simulink model "a2024_V2X_6V_Simulink_model"  (R2023b)
settings: Solver=VariableStepAuto  StartTime=0.0  StopTime=30  MaxStep=1e-2  RelTol=1e-3  AbsTol=1e-3
values from neighbouring files (symbols this model uses):
  b = 1.6    [a2024_v2x_matlab_6veh.m]
  mEgo = 1500    [a2024_v2x_matlab_6veh.m]
  Mode = 1    [a2024_v2x_matlab_6veh.m]    (also in v2x_matlab.m; v2x_matlabV2.m; v2x_matlab_6veh.m; v2x_matlab_R.m)
  pilot = (randi(s,[0 1],pilotsPerSym,1)-0.5)*2    [v2x_matlab.m]
  RxPowerV1 = zeros(sizeEgoWP+2, sizeV1WP+2)    [a2024_v2x_matlab_6veh.m]
  RxPowerV2 = zeros(sizeEgoWP+2, sizeV2WP+2)    [a2024_v2x_matlab_6veh.m]
  RxPowerV3 = zeros(sizeEgoWP+2, sizeV3WP+2)    [a2024_v2x_matlab_6veh.m]
  RxPowerV4 = zeros(sizeEgoWP+2, sizeV4WP+2)    [a2024_v2x_matlab_6veh.m]
  RxPowerV5 = zeros(sizeEgoWP+2, sizeV5WP+2)    [a2024_v2x_matlab_6veh.m]
  RxPowerV6 = zeros(sizeEgoWP+2, sizeV6WP+2)    [a2024_v2x_matlab_6veh.m]
  sampleTime = 0.1    [a2024_v2x_matlab_6veh.m]    (also in v2x_matlab.m; v2x_matlabV2.m; v2x_matlab_6veh.m; v2x_matlab_R.m)
  t_gap = 1.4    [a2024_v2x_matlab_6veh.m]
  waypoints = [egoWP(:,2) egoWP(:,1), zeroforwp]    [a2024_v2x_matlab_6veh.m]    (also in misc.m = data.data.ActorSpecifications(1,1).Waypoints(:,[1,2]); v2x_matlab.m = data.data.ActorSpecifications(1,1).Waypoints(:,[1,2]); v2x_matlabV2.m = [5 -1.6 0; v2x_matlab_R.m = [5 -1.6 0)
  ZeroActors = struct(     'ActorID',0,     'Position', [1000 1000 1000],      'Velocity', [0 0 0],      'Roll', 0,      'Pitch', 0,      'Yaw', 0,      'AngularVelocity', [0 0 0])    [v2x_matlabV2.m]    (also in v2x_matlab_R.m)
undefined symbols (not defined in the file or in its folder): driving, PredictionHorizon, Ts
libraries: commofdm x50, commcnvcod2 x39, simulink x34, commdigbbndam3 x31, commblkintrlv2 x26, commdigbbndpm3 x14, simulink_extras x12, drivingscenarioandsensors x3, mpcadaslib x2, commchan3 x1, vehdynlibdriver x1, commrandsrc3 x1
(part 3 of 6)

== system a2024_V2X_6V_Simulink_model/Subsystem/1//2 64 QAM ==
  Bits : Inport
  Pilot : Inport  Port=2
  Constant2 : Constant  Value=[zeros(887,1)]  VectorParams1D=off  SampleTime=-1
  Convolutional Encoder : commcnvcod2/Convolutional Encoder  trellis=poly2trellis(7, [171 133])  opMode=Truncated (reset every frame)  DelayedResetAction=on  hasIniStPort=off  hasFinStPort=off  usePuncVector=off  punctureVector=[1;1;0;1;1;0;1;1;0;1;0;1;1;0;1;1;0;1]  reset=Unused parameter value
      settings: LibrarySourceBlock=|
      | commhdlcnvcod/Convolutional
      | Encoder
  Display : Display
  OFDM Modulator1 : commofdm/OFDM Modulator  StatePerturbationForJacobian=1.0e-05  FFTLength=1024  NumGuardBandCarriers=[0;0]  InsertDCNull=on  PilotInputPort=on  PilotCarrierIndices=pilotInd  CyclicPrefixLength=512  Windowing=off  WindowLength=16  OversamplingFactor=1  NumSymbols=1  NumTransmitAntennas=1  SimulateUsing=Interpreted execution
  Rectangular QAM Modulator Baseband2 : commdigbbndam3/Rectangular QAM Modulator Baseband  M=2^6  InType=Bit  Enc=Gray  Mapping=[0:15]  PowType=Average Power  MinDist=2  AvgPow=42  PeakPow=1  Ph=0  outDtype=double  outWordLen=16  outUDDataType=sfix(16)  outFracLenMode=Best precision  outFracLen=15  outDataTypeStr=double  outLastDataTypeStr=double
      settings: LibrarySourceBlock=|
      | commhdldigbbndam/Rectangular QAM
      | Modulator
      | Baseband
  Vector Concatenate : Concatenate
  Modulated : Outport
  wires:
  Bits/1 -> Convolutional Encoder/1  "Raw"
  Vector Concatenate/1 -> OFDM Modulator1/1  "After QAM Mod"
  Constant2/1 -> Vector Concatenate/2
  Convolutional Encoder/1 -> Rectangular QAM Modulator Baseband2/1, Display/1  "Before QAM"
  OFDM Modulator1/1 -> Modulated/1  "Sent"
  Pilot/1 -> OFDM Modulator1/2
  Rectangular QAM Modulator Baseband2/1 -> Vector Concatenate/1  "Before OFDM"

== system a2024_V2X_6V_Simulink_model/Subsystem/1//2 QPSK ==
  Bits : Inport
  Pilot : Inport  Port=2
  Constant2 : Constant  Commented=on  Value=[zeros(695,1)]  VectorParams1D=off  SampleTime=-1
  Convolutional Encoder : commcnvcod2/Convolutional Encoder  trellis=poly2trellis(7, [171 133])  opMode=Truncated (reset every frame)  DelayedResetAction=on  hasIniStPort=off  hasFinStPort=off  usePuncVector=on  punctureVector=[1;1]  reset=Unused parameter value
      settings: LibrarySourceBlock=|
      | commhdlcnvcod/Convolutional
      | Encoder
  Gain : Gain  Gain=1/sqrt(10)
  Matrix Concatenate : Concatenate  NumInputs=6  Mode=Multidimensional array  ConcatenateDimension=2
  OFDM Modulator1 : commofdm/OFDM Modulator  StatePerturbationForJacobian=1.0e-05  FFTLength=64  NumGuardBandCarriers=[6;5]  InsertDCNull=on  PilotInputPort=on  PilotCarrierIndices=[12; 26; 40; 54]  CyclicPrefixLength=16  Windowing=off  WindowLength=16  OversamplingFactor=1  NumSymbols=6  NumTransmitAntennas=1  SimulateUsing=Interpreted execution
  QPSK Modulator Baseband : commdigbbndpm3/QPSK Modulator Baseband  InType=Bit  Enc=Gray  Ph=pi/4  outDtype=double  outWordLen=16  outUDDataType=sfix(16)  outFracLenMode=Best precision  outFracLen=15  outDataTypeStr=double  outLastDataTypeStr=double
      settings: LibrarySourceBlock=|
      | commhdldigbbndpm/QPSK
      | Modulator
      | Baseband
  Random Interleaver : commblkintrlv2/Random Interleaver  StatePerturbationForJacobian=1.0e-05  N=576  seed=12345
  Reshape : Reshape  OutputDimensionality=Customize  OutputDimensions=[48,6]
  Vector Concatenate : Concatenate  Commented=on
  Modulated : Outport
  wires:
  OFDM Modulator1/1 -> Modulated/1  "OFDM modulated"
  QPSK Modulator Baseband/1 -> Gain/1
  Bits/1 -> Convolutional Encoder/1
  Convolutional Encoder/1 -> Random Interleaver/1
  Gain/1 -> Reshape/1  "After QAM Mod"
  Pilot/1 -> Matrix Concatenate/1, Matrix Concatenate/2, Matrix Concatenate/3, Matrix Concatenate/6, Matrix Concatenate/5, Matrix Concatenate/4
  Random Interleaver/1 -> QPSK Modulator Baseband/1
  Reshape/1 -> OFDM Modulator1/1
  Constant2/1 -> Vector Concatenate/2
  Matrix Concatenate/1 -> OFDM Modulator1/2

== system a2024_V2X_6V_Simulink_model/Subsystem/3//4 64 QAM ==
  Bits : Inport
  Pilot : Inport  Port=2
  Constant2 : Constant  Value=[zeros(32,1)']  VectorParams1D=off  SampleTime=-1
  Convolutional Encoder : commcnvcod2/Convolutional Encoder  trellis=poly2trellis(7, [171 133])  opMode=Truncated (reset every frame)  DelayedResetAction=on  hasIniStPort=off  hasFinStPort=off  usePuncVector=on  punctureVector=[1;1;0;1;1;0]  reset=Unused parameter value
      settings: LibrarySourceBlock=|
      | commhdlcnvcod/Convolutional
      | Encoder
  Display : Display
  Matrix Concatenate : Concatenate  Mode=Multidimensional array  ConcatenateDimension=2
  OFDM Modulator1 : commofdm/OFDM Modulator  StatePerturbationForJacobian=1.0e-05  FFTLength=64  NumGuardBandCarriers=[6;5]  InsertDCNull=on  PilotInputPort=on  PilotCarrierIndices=[12; 26; 40; 54]  CyclicPrefixLength=16  Windowing=off  WindowLength=16  OversamplingFactor=1  NumSymbols=2  NumTransmitAntennas=1  SimulateUsing=Interpreted execution
  Random Interleaver : commblkintrlv2/Random Interleaver  StatePerturbationForJacobian=1.0e-05  N=384  seed=12345
  Rectangular QAM Modulator Baseband2 : commdigbbndam3/Rectangular QAM Modulator Baseband  M=2^6  InType=Bit  Enc=Gray  Mapping=[0:15]  PowType=Average Power  MinDist=2  AvgPow=0.1  PeakPow=1  Ph=0  outDtype=double  outWordLen=16  outUDDataType=sfix(16)  outFracLenMode=Best precision  outFracLen=15  outDataTypeStr=double  outLastDataTypeStr=double
      settings: LibrarySourceBlock=|
      | commhdldigbbndam/Rectangular QAM
      | Modulator
      | Baseband
  Reshape : Reshape  OutputDimensionality=Customize  OutputDimensions=[48,2]
  Vector Concatenate : Concatenate
  Modulated : Outport
  wires:
  Rectangular QAM Modulator Baseband2/1 -> Vector Concatenate/1  "Before OFDM"
  OFDM Modulator1/1 -> Modulated/1  "Sent"
  Convolutional Encoder/1 -> Random Interleaver/1  "Before QAM"
  Constant2/1 -> Vector Concatenate/2
  Vector Concatenate/1 -> Reshape/1  "After QAM Mod"
  Bits/1 -> Convolutional Encoder/1  "Raw"
  Random Interleaver/1 -> Display/1, Rectangular QAM Modulator Baseband2/1
  Reshape/1 -> OFDM Modulator1/1
  Pilot/1 -> Matrix Concatenate/1, Matrix Concatenate/2
  Matrix Concatenate/1 -> OFDM Modulator1/2

== system a2024_V2X_6V_Simulink_model/Subsystem10/1//2 64 QAM1 ==
  Output : Inport
  Bit to Integer Converter2 : simulink/Logic and Bit Operations/Bit to Integer Converter  nbits=16  bitOrder=MSB first  signedOutputValues=Signed  outDtype=int16  outDtypeSigned=int16
  Complex to Real-Imag : ComplexToRealImag
  Display : Display
  Display2 : Display
  OFDM Demodulator : commofdm/OFDM Demodulator  StatePerturbationForJacobian=1.0e-05  FFTLength=1024  NumGuardBandCarriers=[0; 0]  RemoveDCCarrier=on  PilotOutputPort=on  PilotCarrierIndices=pilotInd  CyclicPrefixLength=512  OversamplingFactor=1  NumSymbols=1  NumReceiveAntennas=1  SimulateUsing=Interpreted execution
  Rectangular QAM Demodulator Baseband2 : commdigbbndam3/Rectangular QAM Demodulator Baseband  M=64  OutType=Bit  DecType=Hard decision  VarSource=Dialog  Variance=1  Dec=Gray  Mapping=[0:15]  PowType=Average Power  MinDist=2  AvgPow=42  PeakPow=1  Ph=0  outDtype1=int16  outDtype2=int16  derotateFactorWordLen=16  derotateFactorDataTypeStr=Inherit: Same word length as input  derotateFactorLastDataTypeStr=Inherit: Same word length as input  denormFactorWordLen=16  denormFactorDataTypeStr=Inherit: Same word length as input  denormFactorLastDataTypeStr=Inherit: Same word length as input  prodOutWordLen=32  prodOutOverflowMode=Wrap  prodOutRoundingMode=Floor  prodOutOvFlMode=off  prodOutOvFlModeLastStrValue=off  sumWordLen=32
      settings: LibrarySourceBlock=|
      | commhdldigbbndam/Rectangular QAM
      | Demodulator
      | Baseband
  Selector : Selector  InputPortWidth=983  IndexOptions=Index vector (dialog)  Indices=[1:96]  OutputSizes=1
  Selector1 : Selector  Commented=on  InputPortWidth=18  IndexOptions=Index vector (dialog)  Indices=[7:18]  OutputSizes=1
  Selector2 : Selector  Commented=on  InputPortWidth=18  IndexOptions=Index vector (dialog)  Indices=[1:6]  OutputSizes=1
  Vector Concatenate : Concatenate  Commented=on
  Viterbi Decoder : commcnvcod2/Viterbi Decoder  trellis=poly2trellis(7, [171 133])  isPunctured=off  punctureVector=[1;1;0;1;1;0;1;1;0;1;0;1;1;0;1;1;0;1]  erasures=off  dectype=Hard decision  nsdecb=4  runSigValErrCheck=off  tbdepth=96  opmode=Truncated  reset=off  delayedResetAction=on  smWordLength=16  outDataType=int16
      settings: LibrarySourceBlock=commhdlcnvcod/Viterbi Decoder
  Modulated : Outport
  wires:
  OFDM Demodulator/2 -> Complex to Real-Imag/1
  Output/1 -> OFDM Demodulator/1  "Sent"
  Selector/1 -> Rectangular QAM Demodulator Baseband2/1  "After OFDM"
  Viterbi Decoder/1 -> Bit to Integer Converter2/1  "Raw"
  OFDM Demodulator/1 -> Selector/1  "After OFDM"
  Rectangular QAM Demodulator Baseband2/1 -> Viterbi Decoder/1  "After QAM"
  Complex to Real-Imag/1 -> Display/1
  Bit to Integer Converter2/1 -> Display2/1, Modulated/1
  Selector1/1 -> Vector Concatenate/1
  Selector2/1 -> Vector Concatenate/2

== system a2024_V2X_6V_Simulink_model/Subsystem10/1//2 QPSK ==
  Output : Inport
  Bit to Integer Converter2 : simulink/Logic and Bit Operations/Bit to Integer Converter  nbits=16  bitOrder=MSB first  signedOutputValues=Signed  outDtype=int16  outDtypeSigned=int16
  Display : Display
  OFDM Demodulator1 : commofdm/OFDM Demodulator  Commented=on  StatePerturbationForJacobian=1.0e-05  FFTLength=64  NumGuardBandCarriers=[0; 0]  RemoveDCCarrier=on  PilotOutputPort=on  PilotCarrierIndices=[12; 26; 40; 54]  CyclicPrefixLength=32  OversamplingFactor=3  NumSymbols=1  NumReceiveAntennas=1  SimulateUsing=Interpreted execution
  OFDM Demodulator2 : commofdm/OFDM Demodulator  StatePerturbationForJacobian=1.0e-05  FFTLength=64  NumGuardBandCarriers=[6; 5]  RemoveDCCarrier=on  PilotOutputPort=on  PilotCarrierIndices=[12; 26; 40; 54]  CyclicPrefixLength=16  OversamplingFactor=1  NumSymbols=6  NumReceiveAntennas=1  SimulateUsing=Interpreted execution
  QPSK Demodulator Baseband : commdigbbndpm3/QPSK Demodulator Baseband  OutType=Bit  DecType=Hard decision  VarSource=Dialog  Variance=1  Dec=Gray  Ph=pi/4  outDtype1=Inherit via internal rule  outDtype2=Inherit via internal rule  derotateFactorWordLen=16  derotateFactorDataTypeStr=Inherit: Same word length as input  derotateFactorLastDataTypeStr=Inherit: Same word length as input
      settings: LibrarySourceBlock=|
      | commhdldigbbndpm/QPSK
      | Demodulator
      | Baseband
  Random Deinterleaver : commblkintrlv2/Random Deinterleaver  StatePerturbationForJacobian=1.0e-05  N=576  seed=12345
  Reshape : Reshape
  Selector : Selector  InputPortWidth=288  IndexOptions=Index vector (dialog)  Indices=[1:288]  OutputSizes=1
  Viterbi Decoder : commcnvcod2/Viterbi Decoder  trellis=poly2trellis(7, [171 133])  isPunctured=on  punctureVector=[1; 1]  erasures=off  dectype=Hard decision  nsdecb=4  runSigValErrCheck=off  tbdepth=30  opmode=Truncated  reset=off  delayedResetAction=on  smWordLength=16  outDataType=Smallest unsigned integer
      settings: LibrarySourceBlock=commhdlcnvcod/Viterbi Decoder
  Modulated : Outport
  wires:
  Random Deinterleaver/1 -> Viterbi Decoder/1
  Reshape/1 -> Selector/1
  Viterbi Decoder/1 -> Bit to Integer Converter2/1
  Bit to Integer Converter2/1 -> Modulated/1
  Selector/1 -> QPSK Demodulator Baseband/1
  QPSK Demodulator Baseband/1 -> Random Deinterleaver/1
  Output/1 -> OFDM Demodulator2/1
  OFDM Demodulator2/1 -> Reshape/1  "Before QAM Demod"
  OFDM Demodulator2/2 -> Display/1

== system a2024_V2X_6V_Simulink_model/Subsystem10/3//4 64 QAM ==
  Output : Inport
  Bit to Integer Converter2 : simulink/Logic and Bit Operations/Bit to Integer Converter  nbits=16  bitOrder=MSB first  signedOutputValues=Signed  outDtype=int16  outDtypeSigned=int16
  Complex to Real-Imag : ComplexToRealImag
  Display : Display
  Display1 : Display
  Display2 : Display
  OFDM Demodulator : commofdm/OFDM Demodulator  StatePerturbationForJacobian=1.0e-05  FFTLength=64  NumGuardBandCarriers=[6; 5]  RemoveDCCarrier=on  PilotOutputPort=on  PilotCarrierIndices=[12; 26; 40; 54]  CyclicPrefixLength=16  OversamplingFactor=1  NumSymbols=2  NumReceiveAntennas=1  SimulateUsing=Interpreted execution
  Random Deinterleaver : commblkintrlv2/Random Deinterleaver  StatePerturbationForJacobian=1.0e-05  N=384  seed=12345
  Rectangular QAM Demodulator Baseband2 : commdigbbndam3/Rectangular QAM Demodulator Baseband  M=64  OutType=Bit  DecType=Hard decision  VarSource=Dialog  Variance=1  Dec=Gray  Mapping=[0:15]  PowType=Average Power  MinDist=2  AvgPow=0.1  PeakPow=1  Ph=0  outDtype1=int16  outDtype2=int16  derotateFactorWordLen=16  derotateFactorDataTypeStr=Inherit: Same word length as input  derotateFactorLastDataTypeStr=Inherit: Same word length as input  denormFactorWordLen=16  denormFactorDataTypeStr=Inherit: Same word length as input  denormFactorLastDataTypeStr=Inherit: Same word length as input  prodOutWordLen=32  prodOutOverflowMode=Wrap  prodOutRoundingMode=Floor  prodOutOvFlMode=off  prodOutOvFlModeLastStrValue=off  sumWordLen=32
      settings: LibrarySourceBlock=|
      | commhdldigbbndam/Rectangular QAM
      | Demodulator
      | Baseband
  Reshape : Reshape
  Selector : Selector  InputPortWidth=96  IndexOptions=Index vector (dialog)  Indices=[1:64]  OutputSizes=1
  Selector1 : Selector  Commented=on  InputPortWidth=18  IndexOptions=Index vector (dialog)  Indices=[7:18]  OutputSizes=1
  Selector2 : Selector  Commented=on  InputPortWidth=18  IndexOptions=Index vector (dialog)  Indices=[1:6]  OutputSizes=1
  Vector Concatenate : Concatenate  Commented=on
  Viterbi Decoder : commcnvcod2/Viterbi Decoder  trellis=poly2trellis(7, [171 133])  isPunctured=on  punctureVector=[1;1;0;1;1;0]  erasures=off  dectype=Hard decision  nsdecb=4  runSigValErrCheck=off  tbdepth=60  opmode=Truncated  reset=off  delayedResetAction=on  smWordLength=16  outDataType=int16
      settings: LibrarySourceBlock=commhdlcnvcod/Viterbi Decoder
  Modulated : Outport
  wires:
  Complex to Real-Imag/2 -> Display1/1
  Random Deinterleaver/1 -> Viterbi Decoder/1
  Reshape/1 -> Selector/1
  Selector2/1 -> Vector Concatenate/2
  Selector1/1 -> Vector Concatenate/1
  Bit to Integer Converter2/1 -> Modulated/1, Display2/1
  Complex to Real-Imag/1 -> Display/1
  Rectangular QAM Demodulator Baseband2/1 -> Random Deinterleaver/1  "After QAM"
  OFDM Demodulator/1 -> Reshape/1  "After OFDM"
  Viterbi Decoder/1 -> Bit to Integer Converter2/1  "Raw"
  Selector/1 -> Rectangular QAM Demodulator Baseband2/1  "After OFDM"
  Output/1 -> OFDM Demodulator/1  "Sent"
  OFDM Demodulator/2 -> Complex to Real-Imag/1

== system a2024_V2X_6V_Simulink_model/Subsystem11/1//2 64 QAM1 ==
  Output : Inport
  Bit to Integer Converter2 : simulink/Logic and Bit Operations/Bit to Integer Converter  nbits=16  bitOrder=MSB first  signedOutputValues=Signed  outDtype=int16  outDtypeSigned=int16
  Complex to Real-Imag : ComplexToRealImag
  Display : Display
  Display2 : Display
  OFDM Demodulator : commofdm/OFDM Demodulator  StatePerturbationForJacobian=1.0e-05  FFTLength=1024  NumGuardBandCarriers=[0; 0]  RemoveDCCarrier=on  PilotOutputPort=on  PilotCarrierIndices=pilotInd  CyclicPrefixLength=512  OversamplingFactor=1  NumSymbols=1  NumReceiveAntennas=1  SimulateUsing=Interpreted execution
  Rectangular QAM Demodulator Baseband2 : commdigbbndam3/Rectangular QAM Demodulator Baseband  M=64  OutType=Bit  DecType=Hard decision  VarSource=Dialog  Variance=1  Dec=Gray  Mapping=[0:15]  PowType=Average Power  MinDist=2  AvgPow=42  PeakPow=1  Ph=0  outDtype1=int16  outDtype2=int16  derotateFactorWordLen=16  derotateFactorDataTypeStr=Inherit: Same word length as input  derotateFactorLastDataTypeStr=Inherit: Same word length as input  denormFactorWordLen=16  denormFactorDataTypeStr=Inherit: Same word length as input  denormFactorLastDataTypeStr=Inherit: Same word length as input  prodOutWordLen=32  prodOutOverflowMode=Wrap  prodOutRoundingMode=Floor  prodOutOvFlMode=off  prodOutOvFlModeLastStrValue=off  sumWordLen=32
      settings: LibrarySourceBlock=|
      | commhdldigbbndam/Rectangular QAM
      | Demodulator
      | Baseband
  Selector : Selector  InputPortWidth=983  IndexOptions=Index vector (dialog)  Indices=[1:96]  OutputSizes=1
  Selector1 : Selector  Commented=on  InputPortWidth=18  IndexOptions=Index vector (dialog)  Indices=[7:18]  OutputSizes=1
  Selector2 : Selector  Commented=on  InputPortWidth=18  IndexOptions=Index vector (dialog)  Indices=[1:6]  OutputSizes=1
  Vector Concatenate : Concatenate  Commented=on
  Viterbi Decoder : commcnvcod2/Viterbi Decoder  trellis=poly2trellis(7, [171 133])  isPunctured=off  punctureVector=[1;1;0;1;1;0;1;1;0;1;0;1;1;0;1;1;0;1]  erasures=off  dectype=Hard decision  nsdecb=4  runSigValErrCheck=off  tbdepth=96  opmode=Truncated  reset=off  delayedResetAction=on  smWordLength=16  outDataType=int16
      settings: LibrarySourceBlock=commhdlcnvcod/Viterbi Decoder
  Modulated : Outport
  wires:
  Selector2/1 -> Vector Concatenate/2
  Selector1/1 -> Vector Concatenate/1
  Bit to Integer Converter2/1 -> Modulated/1, Display2/1
  Complex to Real-Imag/1 -> Display/1
  Rectangular QAM Demodulator Baseband2/1 -> Viterbi Decoder/1  "After QAM"
  OFDM Demodulator/1 -> Selector/1  "After OFDM"
  Viterbi Decoder/1 -> Bit to Integer Converter2/1  "Raw"
  Selector/1 -> Rectangular QAM Demodulator Baseband2/1  "After OFDM"
  Output/1 -> OFDM Demodulator/1  "Sent"
  OFDM Demodulator/2 -> Complex to Real-Imag/1

== system a2024_V2X_6V_Simulink_model/Subsystem11/1//2 QPSK ==
  Output : Inport
  Bit to Integer Converter2 : simulink/Logic and Bit Operations/Bit to Integer Converter  nbits=16  bitOrder=MSB first  signedOutputValues=Signed  outDtype=int16  outDtypeSigned=int16
  Display : Display
  OFDM Demodulator1 : commofdm/OFDM Demodulator  Commented=on  StatePerturbationForJacobian=1.0e-05  FFTLength=64  NumGuardBandCarriers=[0; 0]  RemoveDCCarrier=on  PilotOutputPort=on  PilotCarrierIndices=[12; 26; 40; 54]  CyclicPrefixLength=32  OversamplingFactor=3  NumSymbols=1  NumReceiveAntennas=1  SimulateUsing=Interpreted execution
  OFDM Demodulator2 : commofdm/OFDM Demodulator  StatePerturbationForJacobian=1.0e-05  FFTLength=64  NumGuardBandCarriers=[6; 5]  RemoveDCCarrier=on  PilotOutputPort=on  PilotCarrierIndices=[12; 26; 40; 54]  CyclicPrefixLength=16  OversamplingFactor=1  NumSymbols=6  NumReceiveAntennas=1  SimulateUsing=Interpreted execution
  QPSK Demodulator Baseband : commdigbbndpm3/QPSK Demodulator Baseband  OutType=Bit  DecType=Hard decision  VarSource=Dialog  Variance=1  Dec=Gray  Ph=pi/4  outDtype1=Inherit via internal rule  outDtype2=Inherit via internal rule  derotateFactorWordLen=16  derotateFactorDataTypeStr=Inherit: Same word length as input  derotateFactorLastDataTypeStr=Inherit: Same word length as input
      settings: LibrarySourceBlock=|
      | commhdldigbbndpm/QPSK
      | Demodulator
      | Baseband
  Random Deinterleaver : commblkintrlv2/Random Deinterleaver  StatePerturbationForJacobian=1.0e-05  N=576  seed=12345
  Reshape : Reshape
  Selector : Selector  InputPortWidth=288  IndexOptions=Index vector (dialog)  Indices=[1:288]  OutputSizes=1
  Viterbi Decoder : commcnvcod2/Viterbi Decoder  trellis=poly2trellis(7, [171 133])  isPunctured=on  punctureVector=[1; 1]  erasures=off  dectype=Hard decision  nsdecb=4  runSigValErrCheck=off  tbdepth=30  opmode=Truncated  reset=off  delayedResetAction=on  smWordLength=16  outDataType=Smallest unsigned integer
      settings: LibrarySourceBlock=commhdlcnvcod/Viterbi Decoder
  Modulated : Outport
  wires:
  OFDM Demodulator2/2 -> Display/1
  OFDM Demodulator2/1 -> Reshape/1  "Before QAM Demod"
  Output/1 -> OFDM Demodulator2/1
  QPSK Demodulator Baseband/1 -> Random Deinterleaver/1
  Selector/1 -> QPSK Demodulator Baseband/1
  Bit to Integer Converter2/1 -> Modulated/1
  Viterbi Decoder/1 -> Bit to Integer Converter2/1
  Reshape/1 -> Selector/1
  Random Deinterleaver/1 -> Viterbi Decoder/1

== system a2024_V2X_6V_Simulink_model/Subsystem11/3//4 64 QAM ==
  Output : Inport
  Bit to Integer Converter2 : simulink/Logic and Bit Operations/Bit to Integer Converter  nbits=16  bitOrder=MSB first  signedOutputValues=Signed  outDtype=int16  outDtypeSigned=int16
  Complex to Real-Imag : ComplexToRealImag
  Display : Display
  Display1 : Display
  Display2 : Display
  OFDM Demodulator : commofdm/OFDM Demodulator  StatePerturbationForJacobian=1.0e-05  FFTLength=64  NumGuardBandCarriers=[6; 5]  RemoveDCCarrier=on  PilotOutputPort=on  PilotCarrierIndices=[12; 26; 40; 54]  CyclicPrefixLength=16  OversamplingFactor=1  NumSymbols=2  NumReceiveAntennas=1  SimulateUsing=Interpreted execution
  Random Deinterleaver : commblkintrlv2/Random Deinterleaver  StatePerturbationForJacobian=1.0e-05  N=384  seed=12345
  Rectangular QAM Demodulator Baseband2 : commdigbbndam3/Rectangular QAM Demodulator Baseband  M=64  OutType=Bit  DecType=Hard decision  VarSource=Dialog  Variance=1  Dec=Gray  Mapping=[0:15]  PowType=Average Power  MinDist=2  AvgPow=0.1  PeakPow=1  Ph=0  outDtype1=int16  outDtype2=int16  derotateFactorWordLen=16  derotateFactorDataTypeStr=Inherit: Same word length as input  derotateFactorLastDataTypeStr=Inherit: Same word length as input  denormFactorWordLen=16  denormFactorDataTypeStr=Inherit: Same word length as input  denormFactorLastDataTypeStr=Inherit: Same word length as input  prodOutWordLen=32  prodOutOverflowMode=Wrap  prodOutRoundingMode=Floor  prodOutOvFlMode=off  prodOutOvFlModeLastStrValue=off  sumWordLen=32
      settings: LibrarySourceBlock=|
      | commhdldigbbndam/Rectangular QAM
      | Demodulator
      | Baseband
  Reshape : Reshape
  Selector : Selector  InputPortWidth=96  IndexOptions=Index vector (dialog)  Indices=[1:64]  OutputSizes=1
  Selector1 : Selector  Commented=on  InputPortWidth=18  IndexOptions=Index vector (dialog)  Indices=[7:18]  OutputSizes=1
  Selector2 : Selector  Commented=on  InputPortWidth=18  IndexOptions=Index vector (dialog)  Indices=[1:6]  OutputSizes=1
  Vector Concatenate : Concatenate  Commented=on
  Viterbi Decoder : commcnvcod2/Viterbi Decoder  trellis=poly2trellis(7, [171 133])  isPunctured=on  punctureVector=[1;1;0;1;1;0]  erasures=off  dectype=Hard decision  nsdecb=4  runSigValErrCheck=off  tbdepth=60  opmode=Truncated  reset=off  delayedResetAction=on  smWordLength=16  outDataType=int16
      settings: LibrarySourceBlock=commhdlcnvcod/Viterbi Decoder
  Modulated : Outport
  wires:
  OFDM Demodulator/2 -> Complex to Real-Imag/1
  Output/1 -> OFDM Demodulator/1  "Sent"
  Selector/1 -> Rectangular QAM Demodulator Baseband2/1  "After OFDM"
  Viterbi Decoder/1 -> Bit to Integer Converter2/1  "Raw"
  OFDM Demodulator/1 -> Reshape/1  "After OFDM"
  Rectangular QAM Demodulator Baseband2/1 -> Random Deinterleaver/1  "After QAM"
  Complex to Real-Imag/1 -> Display/1
  Bit to Integer Converter2/1 -> Display2/1, Modulated/1
  Selector1/1 -> Vector Concatenate/1
  Selector2/1 -> Vector Concatenate/2
  Reshape/1 -> Selector/1
  Random Deinterleaver/1 -> Viterbi Decoder/1
  Complex to Real-Imag/2 -> Display1/1

== system a2024_V2X_6V_Simulink_model/Subsystem12/1//2 64 QAM1 ==
  Output : Inport
  Bit to Integer Converter2 : simulink/Logic and Bit Operations/Bit to Integer Converter  nbits=16  bitOrder=MSB first  signedOutputValues=Signed  outDtype=int16  outDtypeSigned=int16
  Complex to Real-Imag : ComplexToRealImag
  Display : Display
  Display2 : Display
  OFDM Demodulator : commofdm/OFDM Demodulator  StatePerturbationForJacobian=1.0e-05  FFTLength=1024  NumGuardBandCarriers=[0; 0]  RemoveDCCarrier=on  PilotOutputPort=on  PilotCarrierIndices=pilotInd  CyclicPrefixLength=512  OversamplingFactor=1  NumSymbols=1  NumReceiveAntennas=1  SimulateUsing=Interpreted execution
  Rectangular QAM Demodulator Baseband2 : commdigbbndam3/Rectangular QAM Demodulator Baseband  M=64  OutType=Bit  DecType=Hard decision  VarSource=Dialog  Variance=1  Dec=Gray  Mapping=[0:15]  PowType=Average Power  MinDist=2  AvgPow=42  PeakPow=1  Ph=0  outDtype1=int16  outDtype2=int16  derotateFactorWordLen=16  derotateFactorDataTypeStr=Inherit: Same word length as input  derotateFactorLastDataTypeStr=Inherit: Same word length as input  denormFactorWordLen=16  denormFactorDataTypeStr=Inherit: Same word length as input  denormFactorLastDataTypeStr=Inherit: Same word length as input  prodOutWordLen=32  prodOutOverflowMode=Wrap  prodOutRoundingMode=Floor  prodOutOvFlMode=off  prodOutOvFlModeLastStrValue=off  sumWordLen=32
      settings: LibrarySourceBlock=|
      | commhdldigbbndam/Rectangular QAM
      | Demodulator
      | Baseband
  Selector : Selector  InputPortWidth=983  IndexOptions=Index vector (dialog)  Indices=[1:96]  OutputSizes=1
  Selector1 : Selector  Commented=on  InputPortWidth=18  IndexOptions=Index vector (dialog)  Indices=[7:18]  OutputSizes=1
  Selector2 : Selector  Commented=on  InputPortWidth=18  IndexOptions=Index vector (dialog)  Indices=[1:6]  OutputSizes=1
  Vector Concatenate : Concatenate  Commented=on
  Viterbi Decoder : commcnvcod2/Viterbi Decoder  trellis=poly2trellis(7, [171 133])  isPunctured=off  punctureVector=[1;1;0;1;1;0;1;1;0;1;0;1;1;0;1;1;0;1]  erasures=off  dectype=Hard decision  nsdecb=4  runSigValErrCheck=off  tbdepth=96  opmode=Truncated  reset=off  delayedResetAction=on  smWordLength=16  outDataType=int16
      settings: LibrarySourceBlock=commhdlcnvcod/Viterbi Decoder
  Modulated : Outport
  wires:
  OFDM Demodulator/2 -> Complex to Real-Imag/1
  Output/1 -> OFDM Demodulator/1  "Sent"
  Selector/1 -> Rectangular QAM Demodulator Baseband2/1  "After OFDM"
  Viterbi Decoder/1 -> Bit to Integer Converter2/1  "Raw"
  OFDM Demodulator/1 -> Selector/1  "After OFDM"
  Rectangular QAM Demodulator Baseband2/1 -> Viterbi Decoder/1  "After QAM"
  Complex to Real-Imag/1 -> Display/1
  Bit to Integer Converter2/1 -> Display2/1, Modulated/1
  Selector1/1 -> Vector Concatenate/1
  Selector2/1 -> Vector Concatenate/2

== system a2024_V2X_6V_Simulink_model/Subsystem12/1//2 QPSK ==
  Output : Inport
  Bit to Integer Converter2 : simulink/Logic and Bit Operations/Bit to Integer Converter  nbits=16  bitOrder=MSB first  signedOutputValues=Signed  outDtype=int16  outDtypeSigned=int16
  Display : Display
  OFDM Demodulator1 : commofdm/OFDM Demodulator  Commented=on  StatePerturbationForJacobian=1.0e-05  FFTLength=64  NumGuardBandCarriers=[0; 0]  RemoveDCCarrier=on  PilotOutputPort=on  PilotCarrierIndices=[12; 26; 40; 54]  CyclicPrefixLength=32  OversamplingFactor=3  NumSymbols=1  NumReceiveAntennas=1  SimulateUsing=Interpreted execution
  OFDM Demodulator2 : commofdm/OFDM Demodulator  StatePerturbationForJacobian=1.0e-05  FFTLength=64  NumGuardBandCarriers=[6; 5]  RemoveDCCarrier=on  PilotOutputPort=on  PilotCarrierIndices=[12; 26; 40; 54]  CyclicPrefixLength=16  OversamplingFactor=1  NumSymbols=6  NumReceiveAntennas=1  SimulateUsing=Interpreted execution
  QPSK Demodulator Baseband : commdigbbndpm3/QPSK Demodulator Baseband  OutType=Bit  DecType=Hard decision  VarSource=Dialog  Variance=1  Dec=Gray  Ph=pi/4  outDtype1=Inherit via internal rule  outDtype2=Inherit via internal rule  derotateFactorWordLen=16  derotateFactorDataTypeStr=Inherit: Same word length as input  derotateFactorLastDataTypeStr=Inherit: Same word length as input
      settings: LibrarySourceBlock=|
      | commhdldigbbndpm/QPSK
      | Demodulator
      | Baseband
  Random Deinterleaver : commblkintrlv2/Random Deinterleaver  StatePerturbationForJacobian=1.0e-05  N=576  seed=12345
  Reshape : Reshape
  Selector : Selector  InputPortWidth=288  IndexOptions=Index vector (dialog)  Indices=[1:288]  OutputSizes=1
  Viterbi Decoder : commcnvcod2/Viterbi Decoder  trellis=poly2trellis(7, [171 133])  isPunctured=on  punctureVector=[1; 1]  erasures=off  dectype=Hard decision  nsdecb=4  runSigValErrCheck=off  tbdepth=30  opmode=Truncated  reset=off  delayedResetAction=on  smWordLength=16  outDataType=Smallest unsigned integer
      settings: LibrarySourceBlock=commhdlcnvcod/Viterbi Decoder
  Modulated : Outport
  wires:
  Random Deinterleaver/1 -> Viterbi Decoder/1
  Reshape/1 -> Selector/1
  Viterbi Decoder/1 -> Bit to Integer Converter2/1
  Bit to Integer Converter2/1 -> Modulated/1
  Selector/1 -> QPSK Demodulator Baseband/1
  QPSK Demodulator Baseband/1 -> Random Deinterleaver/1
  Output/1 -> OFDM Demodulator2/1
  OFDM Demodulator2/1 -> Reshape/1  "Before QAM Demod"
  OFDM Demodulator2/2 -> Display/1

== system a2024_V2X_6V_Simulink_model/Subsystem12/3//4 64 QAM ==
  Output : Inport
  Bit to Integer Converter2 : simulink/Logic and Bit Operations/Bit to Integer Converter  nbits=16  bitOrder=MSB first  signedOutputValues=Signed  outDtype=int16  outDtypeSigned=int16
  Complex to Real-Imag : ComplexToRealImag
  Display : Display
  Display1 : Display
  Display2 : Display
  OFDM Demodulator : commofdm/OFDM Demodulator  StatePerturbationForJacobian=1.0e-05  FFTLength=64  NumGuardBandCarriers=[6; 5]  RemoveDCCarrier=on  PilotOutputPort=on  PilotCarrierIndices=[12; 26; 40; 54]  CyclicPrefixLength=16  OversamplingFactor=1  NumSymbols=2  NumReceiveAntennas=1  SimulateUsing=Interpreted execution
  Random Deinterleaver : commblkintrlv2/Random Deinterleaver  StatePerturbationForJacobian=1.0e-05  N=384  seed=12345
  Rectangular QAM Demodulator Baseband2 : commdigbbndam3/Rectangular QAM Demodulator Baseband  M=64  OutType=Bit  DecType=Hard decision  VarSource=Dialog  Variance=1  Dec=Gray  Mapping=[0:15]  PowType=Average Power  MinDist=2  AvgPow=0.1  PeakPow=1  Ph=0  outDtype1=int16  outDtype2=int16  derotateFactorWordLen=16  derotateFactorDataTypeStr=Inherit: Same word length as input  derotateFactorLastDataTypeStr=Inherit: Same word length as input  denormFactorWordLen=16  denormFactorDataTypeStr=Inherit: Same word length as input  denormFactorLastDataTypeStr=Inherit: Same word length as input  prodOutWordLen=32  prodOutOverflowMode=Wrap  prodOutRoundingMode=Floor  prodOutOvFlMode=off  prodOutOvFlModeLastStrValue=off  sumWordLen=32
      settings: LibrarySourceBlock=|
      | commhdldigbbndam/Rectangular QAM
      | Demodulator
      | Baseband
  Reshape : Reshape
  Selector : Selector  InputPortWidth=96  IndexOptions=Index vector (dialog)  Indices=[1:64]  OutputSizes=1
  Selector1 : Selector  Commented=on  InputPortWidth=18  IndexOptions=Index vector (dialog)  Indices=[7:18]  OutputSizes=1
  Selector2 : Selector  Commented=on  InputPortWidth=18  IndexOptions=Index vector (dialog)  Indices=[1:6]  OutputSizes=1
  Vector Concatenate : Concatenate  Commented=on
  Viterbi Decoder : commcnvcod2/Viterbi Decoder  trellis=poly2trellis(7, [171 133])  isPunctured=on  punctureVector=[1;1;0;1;1;0]  erasures=off  dectype=Hard decision  nsdecb=4  runSigValErrCheck=off  tbdepth=60  opmode=Truncated  reset=off  delayedResetAction=on  smWordLength=16  outDataType=int16
      settings: LibrarySourceBlock=commhdlcnvcod/Viterbi Decoder
  Modulated : Outport
  wires:
  Complex to Real-Imag/2 -> Display1/1
  Random Deinterleaver/1 -> Viterbi Decoder/1
  Reshape/1 -> Selector/1
  Selector2/1 -> Vector Concatenate/2
  Selector1/1 -> Vector Concatenate/1
  Bit to Integer Converter2/1 -> Modulated/1, Display2/1
  Complex to Real-Imag/1 -> Display/1
  Rectangular QAM Demodulator Baseband2/1 -> Random Deinterleaver/1  "After QAM"
  OFDM Demodulator/1 -> Reshape/1  "After OFDM"
  Viterbi Decoder/1 -> Bit to Integer Converter2/1  "Raw"
  Selector/1 -> Rectangular QAM Demodulator Baseband2/1  "After OFDM"
  Output/1 -> OFDM Demodulator/1  "Sent"
  OFDM Demodulator/2 -> Complex to Real-Imag/1

== system a2024_V2X_6V_Simulink_model/Subsystem13/1//2 64 QAM1 ==
  Output : Inport
  Bit to Integer Converter2 : simulink/Logic and Bit Operations/Bit to Integer Converter  nbits=16  bitOrder=MSB first  signedOutputValues=Signed  outDtype=int16  outDtypeSigned=int16
  Complex to Real-Imag : ComplexToRealImag
  Display : Display
  Display2 : Display
  OFDM Demodulator : commofdm/OFDM Demodulator  StatePerturbationForJacobian=1.0e-05  FFTLength=1024  NumGuardBandCarriers=[0; 0]  RemoveDCCarrier=on  PilotOutputPort=on  PilotCarrierIndices=pilotInd  CyclicPrefixLength=512  OversamplingFactor=1  NumSymbols=1  NumReceiveAntennas=1  SimulateUsing=Interpreted execution
  Rectangular QAM Demodulator Baseband2 : commdigbbndam3/Rectangular QAM Demodulator Baseband  M=64  OutType=Bit  DecType=Hard decision  VarSource=Dialog  Variance=1  Dec=Gray  Mapping=[0:15]  PowType=Average Power  MinDist=2  AvgPow=42  PeakPow=1  Ph=0  outDtype1=int16  outDtype2=int16  derotateFactorWordLen=16  derotateFactorDataTypeStr=Inherit: Same word length as input  derotateFactorLastDataTypeStr=Inherit: Same word length as input  denormFactorWordLen=16  denormFactorDataTypeStr=Inherit: Same word length as input  denormFactorLastDataTypeStr=Inherit: Same word length as input  prodOutWordLen=32  prodOutOverflowMode=Wrap  prodOutRoundingMode=Floor  prodOutOvFlMode=off  prodOutOvFlModeLastStrValue=off  sumWordLen=32
      settings: LibrarySourceBlock=|
      | commhdldigbbndam/Rectangular QAM
      | Demodulator
      | Baseband
  Selector : Selector  InputPortWidth=983  IndexOptions=Index vector (dialog)  Indices=[1:96]  OutputSizes=1
  Selector1 : Selector  Commented=on  InputPortWidth=18  IndexOptions=Index vector (dialog)  Indices=[7:18]  OutputSizes=1
  Selector2 : Selector  Commented=on  InputPortWidth=18  IndexOptions=Index vector (dialog)  Indices=[1:6]  OutputSizes=1
  Vector Concatenate : Concatenate  Commented=on
  Viterbi Decoder : commcnvcod2/Viterbi Decoder  trellis=poly2trellis(7, [171 133])  isPunctured=off  punctureVector=[1;1;0;1;1;0;1;1;0;1;0;1;1;0;1;1;0;1]  erasures=off  dectype=Hard decision  nsdecb=4  runSigValErrCheck=off  tbdepth=96  opmode=Truncated  reset=off  delayedResetAction=on  smWordLength=16  outDataType=int16
      settings: LibrarySourceBlock=commhdlcnvcod/Viterbi Decoder
  Modulated : Outport
  wires:
  Selector2/1 -> Vector Concatenate/2
  Selector1/1 -> Vector Concatenate/1
  Bit to Integer Converter2/1 -> Modulated/1, Display2/1
  Complex to Real-Imag/1 -> Display/1
  Rectangular QAM Demodulator Baseband2/1 -> Viterbi Decoder/1  "After QAM"
  OFDM Demodulator/1 -> Selector/1  "After OFDM"
  Viterbi Decoder/1 -> Bit to Integer Converter2/1  "Raw"
  Selector/1 -> Rectangular QAM Demodulator Baseband2/1  "After OFDM"
  Output/1 -> OFDM Demodulator/1  "Sent"
  OFDM Demodulator/2 -> Complex to Real-Imag/1

== system a2024_V2X_6V_Simulink_model/Subsystem13/1//2 QPSK ==
  Output : Inport
  Bit to Integer Converter2 : simulink/Logic and Bit Operations/Bit to Integer Converter  nbits=16  bitOrder=MSB first  signedOutputValues=Signed  outDtype=int16  outDtypeSigned=int16
  Display : Display
  OFDM Demodulator1 : commofdm/OFDM Demodulator  Commented=on  StatePerturbationForJacobian=1.0e-05  FFTLength=64  NumGuardBandCarriers=[0; 0]  RemoveDCCarrier=on  PilotOutputPort=on  PilotCarrierIndices=[12; 26; 40; 54]  CyclicPrefixLength=32  OversamplingFactor=3  NumSymbols=1  NumReceiveAntennas=1  SimulateUsing=Interpreted execution
  OFDM Demodulator2 : commofdm/OFDM Demodulator  StatePerturbationForJacobian=1.0e-05  FFTLength=64  NumGuardBandCarriers=[6; 5]  RemoveDCCarrier=on  PilotOutputPort=on  PilotCarrierIndices=[12; 26; 40; 54]  CyclicPrefixLength=16  OversamplingFactor=1  NumSymbols=6  NumReceiveAntennas=1  SimulateUsing=Interpreted execution
  QPSK Demodulator Baseband : commdigbbndpm3/QPSK Demodulator Baseband  OutType=Bit  DecType=Hard decision  VarSource=Dialog  Variance=1  Dec=Gray  Ph=pi/4  outDtype1=Inherit via internal rule  outDtype2=Inherit via internal rule  derotateFactorWordLen=16  derotateFactorDataTypeStr=Inherit: Same word length as input  derotateFactorLastDataTypeStr=Inherit: Same word length as input
      settings: LibrarySourceBlock=|
      | commhdldigbbndpm/QPSK
      | Demodulator
      | Baseband
  Random Deinterleaver : commblkintrlv2/Random Deinterleaver  StatePerturbationForJacobian=1.0e-05  N=576  seed=12345
  Reshape : Reshape
  Selector : Selector  InputPortWidth=288  IndexOptions=Index vector (dialog)  Indices=[1:288]  OutputSizes=1
  Viterbi Decoder : commcnvcod2/Viterbi Decoder  trellis=poly2trellis(7, [171 133])  isPunctured=on  punctureVector=[1; 1]  erasures=off  dectype=Hard decision  nsdecb=4  runSigValErrCheck=off  tbdepth=30  opmode=Truncated  reset=off  delayedResetAction=on  smWordLength=16  outDataType=Smallest unsigned integer
      settings: LibrarySourceBlock=commhdlcnvcod/Viterbi Decoder
  Modulated : Outport
  wires:
  OFDM Demodulator2/2 -> Display/1
  OFDM Demodulator2/1 -> Reshape/1  "Before QAM Demod"
  Output/1 -> OFDM Demodulator2/1
  QPSK Demodulator Baseband/1 -> Random Deinterleaver/1
  Selector/1 -> QPSK Demodulator Baseband/1
  Bit to Integer Converter2/1 -> Modulated/1
  Viterbi Decoder/1 -> Bit to Integer Converter2/1
  Reshape/1 -> Selector/1
  Random Deinterleaver/1 -> Viterbi Decoder/1

== system a2024_V2X_6V_Simulink_model/Subsystem13/3//4 64 QAM ==
  Output : Inport
  Bit to Integer Converter2 : simulink/Logic and Bit Operations/Bit to Integer Converter  nbits=16  bitOrder=MSB first  signedOutputValues=Signed  outDtype=int16  outDtypeSigned=int16
  Complex to Real-Imag : ComplexToRealImag
  Display : Display
  Display1 : Display
  Display2 : Display
  OFDM Demodulator : commofdm/OFDM Demodulator  StatePerturbationForJacobian=1.0e-05  FFTLength=64  NumGuardBandCarriers=[6; 5]  RemoveDCCarrier=on  PilotOutputPort=on  PilotCarrierIndices=[12; 26; 40; 54]  CyclicPrefixLength=16  OversamplingFactor=1  NumSymbols=2  NumReceiveAntennas=1  SimulateUsing=Interpreted execution
  Random Deinterleaver : commblkintrlv2/Random Deinterleaver  StatePerturbationForJacobian=1.0e-05  N=384  seed=12345
  Rectangular QAM Demodulator Baseband2 : commdigbbndam3/Rectangular QAM Demodulator Baseband  M=64  OutType=Bit  DecType=Hard decision  VarSource=Dialog  Variance=1  Dec=Gray  Mapping=[0:15]  PowType=Average Power  MinDist=2  AvgPow=0.1  PeakPow=1  Ph=0  outDtype1=int16  outDtype2=int16  derotateFactorWordLen=16  derotateFactorDataTypeStr=Inherit: Same word length as input  derotateFactorLastDataTypeStr=Inherit: Same word length as input  denormFactorWordLen=16  denormFactorDataTypeStr=Inherit: Same word length as input  denormFactorLastDataTypeStr=Inherit: Same word length as input  prodOutWordLen=32  prodOutOverflowMode=Wrap  prodOutRoundingMode=Floor  prodOutOvFlMode=off  prodOutOvFlModeLastStrValue=off  sumWordLen=32
      settings: LibrarySourceBlock=|
      | commhdldigbbndam/Rectangular QAM
      | Demodulator
      | Baseband
  Reshape : Reshape
  Selector : Selector  InputPortWidth=96  IndexOptions=Index vector (dialog)  Indices=[1:64]  OutputSizes=1
  Selector1 : Selector  Commented=on  InputPortWidth=18  IndexOptions=Index vector (dialog)  Indices=[7:18]  OutputSizes=1
  Selector2 : Selector  Commented=on  InputPortWidth=18  IndexOptions=Index vector (dialog)  Indices=[1:6]  OutputSizes=1
  Vector Concatenate : Concatenate  Commented=on
  Viterbi Decoder : commcnvcod2/Viterbi Decoder  trellis=poly2trellis(7, [171 133])  isPunctured=on  punctureVector=[1;1;0;1;1;0]  erasures=off  dectype=Hard decision  nsdecb=4  runSigValErrCheck=off  tbdepth=60  opmode=Truncated  reset=off  delayedResetAction=on  smWordLength=16  outDataType=int16
      settings: LibrarySourceBlock=commhdlcnvcod/Viterbi Decoder
  Modulated : Outport
  wires:
  OFDM Demodulator/2 -> Complex to Real-Imag/1
  Output/1 -> OFDM Demodulator/1  "Sent"
  Selector/1 -> Rectangular QAM Demodulator Baseband2/1  "After OFDM"
  Viterbi Decoder/1 -> Bit to Integer Converter2/1  "Raw"
  OFDM Demodulator/1 -> Reshape/1  "After OFDM"
  Rectangular QAM Demodulator Baseband2/1 -> Random Deinterleaver/1  "After QAM"
  Complex to Real-Imag/1 -> Display/1
  Bit to Integer Converter2/1 -> Display2/1, Modulated/1
  Selector1/1 -> Vector Concatenate/1
  Selector2/1 -> Vector Concatenate/2
  Reshape/1 -> Selector/1
  Random Deinterleaver/1 -> Viterbi Decoder/1
  Complex to Real-Imag/2 -> Display1/1

== system a2024_V2X_6V_Simulink_model/Subsystem14/1//2 64 QAM1 ==
  Output : Inport
  Bit to Integer Converter2 : simulink/Logic and Bit Operations/Bit to Integer Converter  nbits=16  bitOrder=MSB first  signedOutputValues=Signed  outDtype=int16  outDtypeSigned=int16
  Complex to Real-Imag : ComplexToRealImag
  Display : Display
  Display2 : Display
  OFDM Demodulator : commofdm/OFDM Demodulator  StatePerturbationForJacobian=1.0e-05  FFTLength=1024  NumGuardBandCarriers=[0; 0]  RemoveDCCarrier=on  PilotOutputPort=on  PilotCarrierIndices=pilotInd  CyclicPrefixLength=512  OversamplingFactor=1  NumSymbols=1  NumReceiveAntennas=1  SimulateUsing=Interpreted execution
  Rectangular QAM Demodulator Baseband2 : commdigbbndam3/Rectangular QAM Demodulator Baseband  M=64  OutType=Bit  DecType=Hard decision  VarSource=Dialog  Variance=1  Dec=Gray  Mapping=[0:15]  PowType=Average Power  MinDist=2  AvgPow=42  PeakPow=1  Ph=0  outDtype1=int16  outDtype2=int16  derotateFactorWordLen=16  derotateFactorDataTypeStr=Inherit: Same word length as input  derotateFactorLastDataTypeStr=Inherit: Same word length as input  denormFactorWordLen=16  denormFactorDataTypeStr=Inherit: Same word length as input  denormFactorLastDataTypeStr=Inherit: Same word length as input  prodOutWordLen=32  prodOutOverflowMode=Wrap  prodOutRoundingMode=Floor  prodOutOvFlMode=off  prodOutOvFlModeLastStrValue=off  sumWordLen=32
      settings: LibrarySourceBlock=|
      | commhdldigbbndam/Rectangular QAM
      | Demodulator
      | Baseband
  Selector : Selector  InputPortWidth=983  IndexOptions=Index vector (dialog)  Indices=[1:96]  OutputSizes=1
  Selector1 : Selector  Commented=on  InputPortWidth=18  IndexOptions=Index vector (dialog)  Indices=[7:18]  OutputSizes=1
  Selector2 : Selector  Commented=on  InputPortWidth=18  IndexOptions=Index vector (dialog)  Indices=[1:6]  OutputSizes=1
  Vector Concatenate : Concatenate  Commented=on
  Viterbi Decoder : commcnvcod2/Viterbi Decoder  trellis=poly2trellis(7, [171 133])  isPunctured=off  punctureVector=[1;1;0;1;1;0;1;1;0;1;0;1;1;0;1;1;0;1]  erasures=off  dectype=Hard decision  nsdecb=4  runSigValErrCheck=off  tbdepth=96  opmode=Truncated  reset=off  delayedResetAction=on  smWordLength=16  outDataType=int16
      settings: LibrarySourceBlock=commhdlcnvcod/Viterbi Decoder
  Modulated : Outport
  wires:
  OFDM Demodulator/2 -> Complex to Real-Imag/1
  Output/1 -> OFDM Demodulator/1  "Sent"
  Selector/1 -> Rectangular QAM Demodulator Baseband2/1  "After OFDM"
  Viterbi Decoder/1 -> Bit to Integer Converter2/1  "Raw"
  OFDM Demodulator/1 -> Selector/1  "After OFDM"
  Rectangular QAM Demodulator Baseband2/1 -> Viterbi Decoder/1  "After QAM"
  Complex to Real-Imag/1 -> Display/1
  Bit to Integer Converter2/1 -> Display2/1, Modulated/1
  Selector1/1 -> Vector Concatenate/1
  Selector2/1 -> Vector Concatenate/2

== system a2024_V2X_6V_Simulink_model/Subsystem14/1//2 QPSK ==
  Output : Inport
  Bit to Integer Converter2 : simulink/Logic and Bit Operations/Bit to Integer Converter  nbits=16  bitOrder=MSB first  signedOutputValues=Signed  outDtype=int16  outDtypeSigned=int16
  Display : Display
  OFDM Demodulator1 : commofdm/OFDM Demodulator  Commented=on  StatePerturbationForJacobian=1.0e-05  FFTLength=64  NumGuardBandCarriers=[0; 0]  RemoveDCCarrier=on  PilotOutputPort=on  PilotCarrierIndices=[12; 26; 40; 54]  CyclicPrefixLength=32  OversamplingFactor=3  NumSymbols=1  NumReceiveAntennas=1  SimulateUsing=Interpreted execution
  OFDM Demodulator2 : commofdm/OFDM Demodulator  StatePerturbationForJacobian=1.0e-05  FFTLength=64  NumGuardBandCarriers=[6; 5]  RemoveDCCarrier=on  PilotOutputPort=on  PilotCarrierIndices=[12; 26; 40; 54]  CyclicPrefixLength=16  OversamplingFactor=1  NumSymbols=6  NumReceiveAntennas=1  SimulateUsing=Interpreted execution
  QPSK Demodulator Baseband : commdigbbndpm3/QPSK Demodulator Baseband  OutType=Bit  DecType=Hard decision  VarSource=Dialog  Variance=1  Dec=Gray  Ph=pi/4  outDtype1=Inherit via internal rule  outDtype2=Inherit via internal rule  derotateFactorWordLen=16  derotateFactorDataTypeStr=Inherit: Same word length as input  derotateFactorLastDataTypeStr=Inherit: Same word length as input
      settings: LibrarySourceBlock=|
      | commhdldigbbndpm/QPSK
      | Demodulator
      | Baseband
  Random Deinterleaver : commblkintrlv2/Random Deinterleaver  StatePerturbationForJacobian=1.0e-05  N=576  seed=12345
  Reshape : Reshape
  Selector : Selector  InputPortWidth=288  IndexOptions=Index vector (dialog)  Indices=[1:288]  OutputSizes=1
  Viterbi Decoder : commcnvcod2/Viterbi Decoder  trellis=poly2trellis(7, [171 133])  isPunctured=on  punctureVector=[1; 1]  erasures=off  dectype=Hard decision  nsdecb=4  runSigValErrCheck=off  tbdepth=30  opmode=Truncated  reset=off  delayedResetAction=on  smWordLength=16  outDataType=Smallest unsigned integer
      settings: LibrarySourceBlock=commhdlcnvcod/Viterbi Decoder
  Modulated : Outport
  wires:
  Random Deinterleaver/1 -> Viterbi Decoder/1
  Reshape/1 -> Selector/1
  Viterbi Decoder/1 -> Bit to Integer Converter2/1
  Bit to Integer Converter2/1 -> Modulated/1
  Selector/1 -> QPSK Demodulator Baseband/1
  QPSK Demodulator Baseband/1 -> Random Deinterleaver/1
  Output/1 -> OFDM Demodulator2/1
  OFDM Demodulator2/1 -> Reshape/1  "Before QAM Demod"
  OFDM Demodulator2/2 -> Display/1
